simulink library "INT_EngBrk_ECRCtl"  (R2016b)
settings: Solver=VariableStepAuto  StartTime=0.0  StopTime=10.0  RelTol=1e-3
settings Model: Creator=lenovo  LastModifiedBy=lenovo

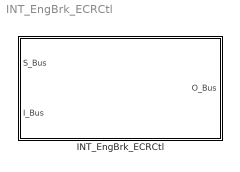
== system INT_EngBrk_ECRCtl ==
  INT_EngBrk_ECRCtl : Subsystem

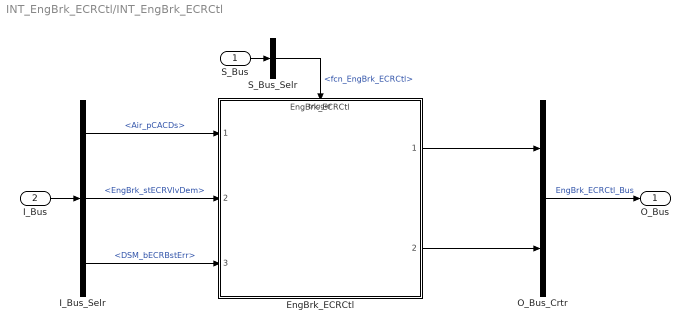
== system INT_EngBrk_ECRCtl/INT_EngBrk_ECRCtl ==
  S_Bus : Inport
  I_Bus : Inport  Port=2
  EngBrk_ECRCtl : ModelReference  ModelNameDialog=EngBrk_ECRCtl  ModelReferenceVersion=1.3  TriggerPortName=function  TriggerPortTriggerType=function-call  TriggerPortStatesWhenEnabling=held
  I_Bus_Selr : BusSelector  OutputSignals=Air_pCACDs,EngBrk_stECRVlvDem,DSM_bECRBstErr
  O_Bus_Crtr : BusCreator  Inputs=2
  S_Bus_Selr : BusSelector  OutputSignals=fcn_EngBrk_ECRCtl
  O_Bus : Outport
  wires:
  S_Bus_Selr/1 -> EngBrk_ECRCtl/Trigger  "<fcn_EngBrk_ECRCtl>"
  S_Bus/1 -> S_Bus_Selr/1
  I_Bus/1 -> I_Bus_Selr/1
  I_Bus_Selr/1 -> EngBrk_ECRCtl/1  "<Air_pCACDs>"
  I_Bus_Selr/2 -> EngBrk_ECRCtl/2  "<EngBrk_stECRVlvDem>"
  I_Bus_Selr/3 -> EngBrk_ECRCtl/3  "<DSM_bECRBstErr>"
  O_Bus_Crtr/1 -> O_Bus/1  "EngBrk_ECRCtl_Bus"
  EngBrk_ECRCtl/1 -> O_Bus_Crtr/1
  EngBrk_ECRCtl/2 -> O_Bus_Crtr/2
